simulink model "gm_motor_dtf_step_fixdt"  (R2021b)
settings: Solver=FixedStepAuto  StartTime=0.0  StopTime=120  FixedStep=0.001  RelTol=1e-3
undefined symbols (not defined in the file or in its folder): DiscIntNeverNeededParam
Description:
  | Symmetric FIR Filter
  | This example shows how to use HDL Coder(TM) to check, generate,
  | and verify HDL for a fixed-point symmetric FIR filter.
settings Model: Creator=The MathWorks, Inc.  LastModifiedBy=Marco Milanesi
settings SolverCC: AlgebraicLoopSolver=TrustRegion  AutoInsertRateTranBlk=on
settings DataIOCC: LimitDataPoints=on  SaveFormat=Array  SaveOutput=off  SignalLogging=off  SaveTime=off  ReturnWorkspaceOutputs=off  SignalLoggingName=logsOut
settings OptimizationCC: BlockReduction=off  BooleanDataType=off  ConditionallyExecuteInputs=off  DefaultParameterBehavior=Inlined  InheritOutputTypeSmallerThanSingle=on  InlineInvariantSignals=on  ExpressionDepthLimit=2147483647  InitFltsAndDblsToZero=on  LifeSpan=inf  BufferReusableBoundary=off
settings DebuggingCC: AlgebraicLoopMsg=error  SaveWithParameterizedLinksMsg=none  UnderspecifiedInitializationDetection=Classic  MergeDetectMultiDrivingBlocksExec=none  CheckExecutionContextPreStartOutputMsg=on  SignalResolutionControl=TryResolveAllWithWarning  InheritedTsInSrcMsg=none  MultiTaskDSMMsg=warning  MultiTaskCondExecSysMsg=none  SingleTaskRateTransMsg=error  IntegerOverflowMsg=none  ParameterPrecisionLossMsg=none  FcnCallInpInsideContextMsg=warning  BusObjectLabelMismatch=none  StateNameClashWarn=warning  SFUnexpectedBacktrackingDiag=warning  SFNoUnconditionalDefaultTransitionDiag=warning  SFExecutionAtInitializationDiag=none  SFMachineParentedDataDiag=warning  IntegerSaturationMsg=none  ArithmeticOperatorsInVariantConditions=warning
settings HardwareCC: ProdBitPerPointer=32  ProdBitPerSizeT=32  ProdBitPerPtrDiffT=32  ProdLargestAtomicFloat=None  ProdIntDivRoundTo=Undefined  ProdEndianess=Unspecified  ProdWordSize=32  ProdHWDeviceType=ASIC/FPGA  TargetUnknown=on  ProdEqTarget=off
settings ModelReferenceCC: PropagateSignalLabelsOutOfModel=off
settings SFSimCC: SimUseLocalCustomCode=off  CustomCodeUndefinedFunction=UseInterfaceOnly
settings RTWCC: RTWUseLocalCustomCode=off
settings CodeAppCC: StateflowObjectComments=on
settings GRTTargetCC: TargetFcnLib=ansi_tfl_tmw.mat  TargetLangStandard=C89/C90 (ANSI)  CombineOutputUpdateFcns=off  GRTInterface=on
settings ConfigComp: CovMetricSettings=dw  CovSaveCumulativeToWorkspaceVar=on  CovSaveSingleToWorkspaceVar=on  CovExternalEMLEnable=off

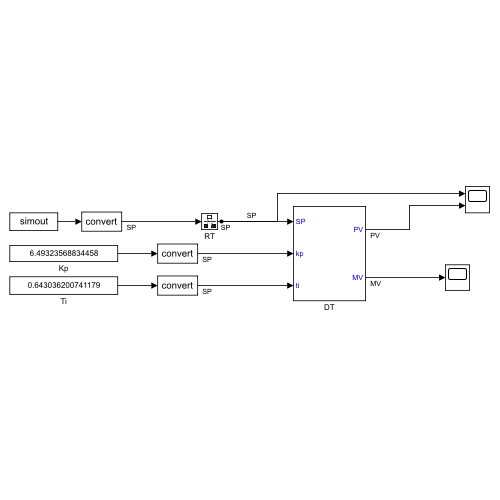
[thumbnail: Simulink's stored preview of the top-level diagram]
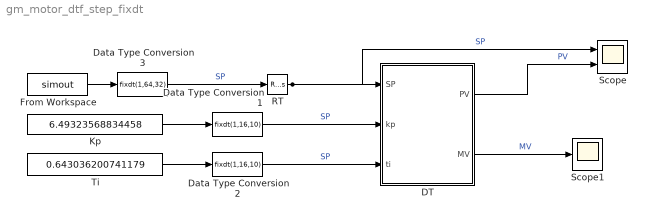
== system gm_motor_dtf_step_fixdt ==
  DT : Subsystem
  Data Type Conversion1 : DataTypeConversion  OutDataTypeStr=fixdt(1,16,10)
  Data Type Conversion2 : DataTypeConversion  OutDataTypeStr=fixdt(1,16,10)
  Data Type Conversion3 : DataTypeConversion  OutDataTypeStr=fixdt(1,64,32)
  From Workspace : FromWorkspace  VariableName=simout  SampleTime=1  OutputAfterFinalValue=Setting to zero
  Kp : Constant  Value=6.49323568834458
  RT : RateTransition  OutPortSampleTime=0.001
  Scope : Scope  NumInputPorts=2
  Scope1 : Scope
  Ti : Constant  Value=0.643036200741179
  wires:
  Data Type Conversion3/1 -> RT/1  "SP"
  DT/1(PV) -> Scope/2  "PV"
  From Workspace/1 -> Data Type Conversion3/1
  Ti/1 -> Data Type Conversion2/1
  Data Type Conversion2/1 -> DT/3(ti)  "SP"
  Data Type Conversion1/1 -> DT/2(kp)  "SP"
  Kp/1 -> Data Type Conversion1/1
  DT/2(MV) -> Scope1/1  "MV"
  RT/1 -> DT/1(SP), Scope/1  "SP"

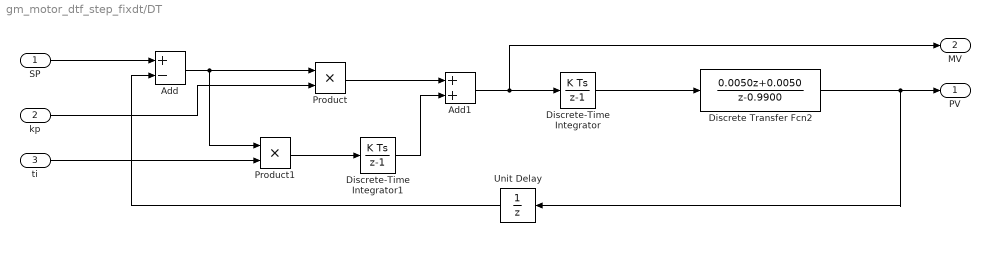
== system gm_motor_dtf_step_fixdt/DT ==
  SP : Inport
  kp : Inport  Port=2
  ti : Inport  Port=3
  Add : Sum  Inputs=+-  AccumDataTypeStr=fixdt(1,64,32)  OutDataTypeStr=fixdt(1,64,32)
  Add1 : Sum  AccumDataTypeStr=fixdt(1,64,32)  OutDataTypeStr=fixdt(1,64,32)
  Discrete Transfer Fcn2 : DiscreteTransferFcn  Numerator=[0.0050 0.0050]  Denominator=[1 -0.9900]  NumCoefDataTypeStr=fixdt(1,64,32)  DenCoefDataTypeStr=fixdt(1,64,32)  NumProductDataTypeStr=fixdt(1,64,32)  DenProductDataTypeStr=fixdt(1,64,32)  NumAccumDataTypeStr=fixdt(1,64,32)  DenAccumDataTypeStr=fixdt(1,64,32)  OutDataTypeStr=fixdt(1,64,32)
  Discrete-Time Integrator : DiscreteIntegrator  SampleTime=-1  OutDataTypeStr=fixdt(1,64,32)  ICPrevOutput=DiscIntNeverNeededParam  ICPrevScaledInput=DiscIntNeverNeededParam
  Discrete-Time Integrator1 : DiscreteIntegrator  SampleTime=0.001  OutDataTypeStr=fixdt(1,64,32)  ICPrevOutput=DiscIntNeverNeededParam  ICPrevScaledInput=DiscIntNeverNeededParam
  Product : Product  OutDataTypeStr=fixdt(1,64,32)
  Product1 : Product  OutDataTypeStr=fixdt(1,64,32)
  Unit Delay : UnitDelay  SampleTime=0.001  HasFrameUpgradeWarning=on
  PV : Outport  VectorParamsAs1DForOutWhenUnconnected=off
  MV : Outport  Port=2  VectorParamsAs1DForOutWhenUnconnected=off
  wires:
  Unit Delay/1 -> Add/2
  Discrete-Time Integrator/1 -> Discrete Transfer Fcn2/1
  Add1/1 -> Discrete-Time Integrator/1, MV/1
  Discrete-Time Integrator1/1 -> Add1/2
  Product1/1 -> Discrete-Time Integrator1/1
  ti/1 -> Product1/2
  Product/1 -> Add1/1
  kp/1 -> Product/2
  Add/1 -> Product1/1, Product/1
  Discrete Transfer Fcn2/1 -> PV/1, Unit Delay/1
  SP/1 -> Add/1
